simulink model "Ex2Week1Sim"  (R2023b)
settings: Solver=VariableStepAuto  StartTime=0.0  StopTime=10.0  RelTol=1e-3
settings Model: Creator=andyjwaideh  LastModifiedBy=andyjwaideh

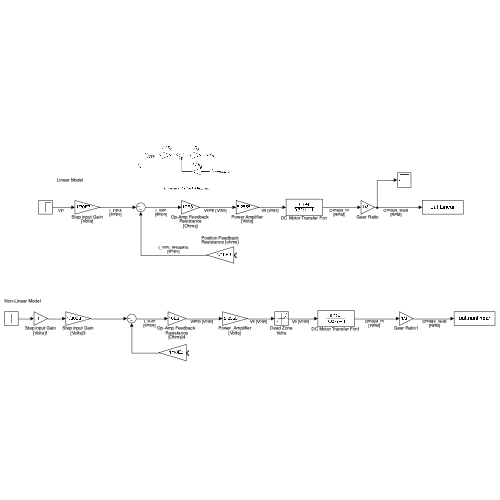
[thumbnail: Simulink's stored preview of the top-level diagram]
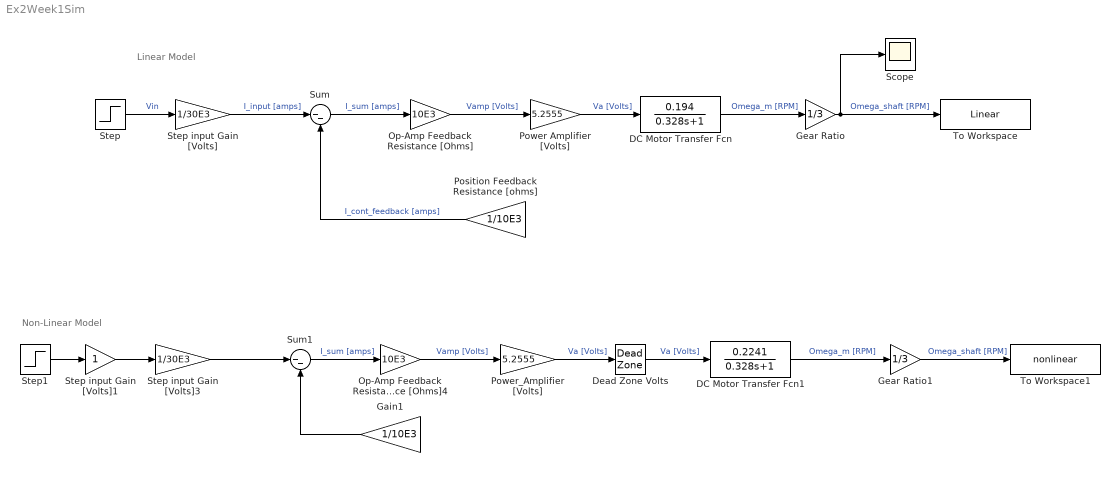
== system Ex2Week1Sim ==
  note: Non-Linear Model
  note: Linear Model
  DC Motor Transfer Fcn : TransferFcn  Numerator=[0.194]  Denominator=[0.328 1]
  DC Motor Transfer Fcn1 : TransferFcn  Numerator=[0.2241]  Denominator=[0.328 1]
  Dead Zone Volts : DeadZone  LowerValue=1  UpperValue=1
  Gain1 : Gain  Gain=1/10E3
  Gear Ratio : Gain  Gain=1/3
  Gear Ratio1 : Gain  Gain=1/3
  Op-Amp Feedback Resistance [Ohms] : Gain  Gain=10E3
  Op-Amp Feedback Resistance [Ohms]4 : Gain  Gain=10E3
  Position Feedback Resistance [ohms] : Gain  Gain=1/10E3
  Power Amplifier [Volts] : Gain  Gain=5.2555
  Power_Amplifier [Volts] : Gain  Gain=5.2555
  Scope : Scope
  Step : Step  SampleTime=0
  Step input Gain [Volts] : Gain  Gain=1/30E3
  Step input Gain [Volts]1 : Gain
  Step input Gain [Volts]3 : Gain  Gain=1/30E3
  Step1 : Step  SampleTime=0
  Sum : Sum  Inputs=|--
  Sum1 : Sum  Inputs=|--
  To Workspace : ToWorkspace  VariableName=Linear  SaveFormat=Timeseries  SampleTime=-1
  To Workspace1 : ToWorkspace  VariableName=nonlinear  SaveFormat=Timeseries  SampleTime=-1
  wires:
  Step1/1 -> Step input Gain [Volts]1/1
  Power Amplifier [Volts]/1 -> DC Motor Transfer Fcn/1  "Va [Volts]"
  DC Motor Transfer Fcn/1 -> Gear Ratio/1  "Omega_m [RPM]"
  Gear Ratio/1 -> Scope/1, To Workspace/1  "Omega_shaft [RPM]"
  DC Motor Transfer Fcn1/1 -> Gear Ratio1/1  "Omega_m [RPM]"
  Power_Amplifier [Volts]/1 -> Dead Zone Volts/1  "Va [Volts]"
  Dead Zone Volts/1 -> DC Motor Transfer Fcn1/1  "Va [Volts]"
  Step/1 -> Step input Gain [Volts]/1  "Vin"
  Step input Gain [Volts]/1 -> Sum/1  "I_input [amps]"
  Op-Amp Feedback Resistance [Ohms]/1 -> Power Amplifier [Volts]/1  "Vamp [Volts]"
  Sum/1 -> Op-Amp Feedback Resistance [Ohms]/1  "I_sum [amps]"
  Position Feedback Resistance [ohms]/1 -> Sum/2  "I_cont_feedback [amps]"
  Gain1/1 -> Sum1/2
  Sum1/1 -> Op-Amp Feedback Resistance [Ohms]4/1  "I_sum [amps]"
  Op-Amp Feedback Resistance [Ohms]4/1 -> Power_Amplifier [Volts]/1  "Vamp [Volts]"
  Step input Gain [Volts]3/1 -> Sum1/1
  Gear Ratio1/1 -> To Workspace1/1  "Omega_shaft [RPM]"
  Step input Gain [Volts]1/1 -> Step input Gain [Volts]3/1
